simulink model "ModeShape_IEEE14_case1"  (R2022b)
settings: Solver=FixedStepAuto  StartTime=0.0  StopTime=15  FixedStep=Ts  RelTol=1e-3
InitFcn:
  | load('data_idq_all');
  | load('data_vdq_all');
  | ModeSel = 151; % case1
  | run Mode_Right_Eig.m;
StartFcn:
  | load('data_idq_all');
  | load('data_vdq_all');
  | ModeSel = 151; % case1
  | run Mode_Right_Eig.m;
values from neighbouring files (symbols this model uses):
  freq_sel = imag(Mode_Hz)    [Mode_Right_Eig.m]
  Mode_Rad = D(ModeSel, ModeSel)    [Mode_Right_Eig.m]
  Phi_vec_trim = Phi_vec_trim.'    [Mode_Right_Eig.m]
  Psi_vec_trim = Psi_vec_trim.'    [Mode_Right_Eig.m]
undefined symbols (not defined in the file or in its folder): Ts
libraries: eeGeneralControl x4, spsPLLLib x1
settings Model: Creator=y_zhu  LastModifiedBy=yz34218

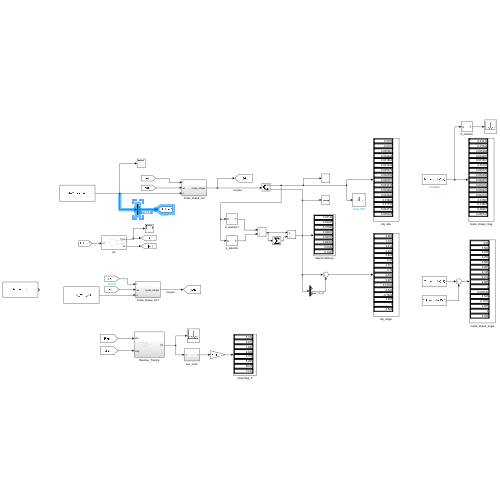
[thumbnail: Simulink's stored preview of the top-level diagram]
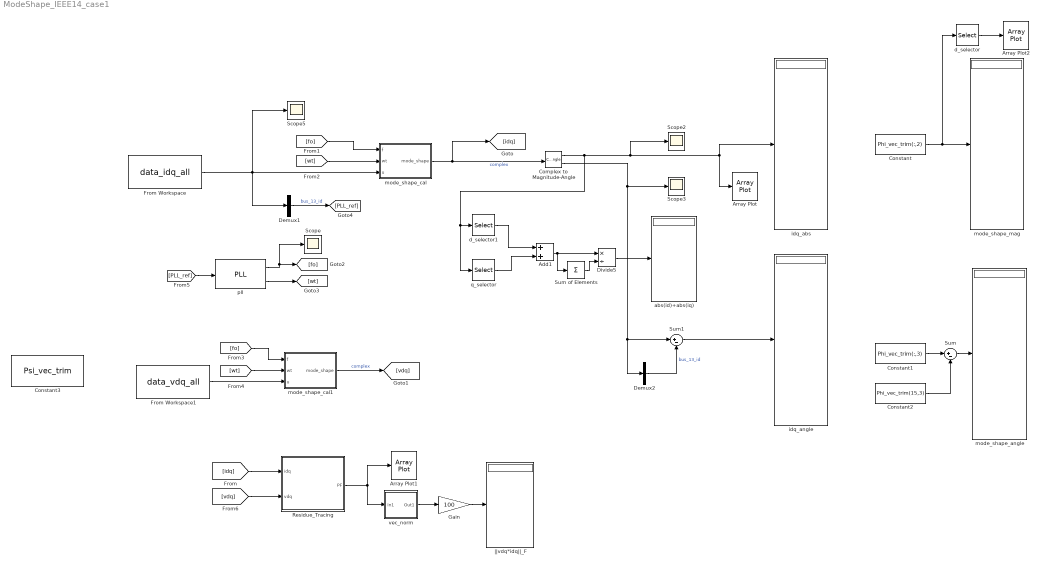
== system ModeShape_IEEE14_case1 ==
  Add1 : Sum
  Array Plot : ArrayPlot  WindowPosition=[-4.000000,155.000000,800.000000,500.000000,]  ScopeFrameLocation=window  YLimits=[-0.001,0.0195]
  Array Plot1 : ArrayPlot  WindowPosition=[913.000000,343.000000,800.000000,500.000000,]  ScopeFrameLocation=window  YLimits=[-0.0628,0.6743]
  Array Plot2 : ArrayPlot  WindowPosition=[402.000000,155.000000,800.000000,621.000000,]  ScopeFrameLocation=window  YLimits=[-0.0001,0.018]
  Complex to Magnitude-Angle : ComplexToMagnitudeAngle
  Constant : Constant  Value=Phi_vec_trim(:,2)
  Constant1 : Constant  Value=Phi_vec_trim(:,3)
  Constant2 : Constant  Value=Phi_vec_trim(15,3)
  Constant3 : Constant  Value=Psi_vec_trim
  Demux1 : Demux  Outputs=[14,1,1]
  Demux2 : Demux  Outputs=[14,1,1]
  Divide5 : Product  Inputs=*/
  From Workspace : FromWorkspace  VariableName=data_idq_all
  From Workspace1 : FromWorkspace  VariableName=data_vdq_all
  Gain : Gain  Gain=100
  Residue_Tracing : Subsystem
  Scope{,2..3,5} (4 alike) : Scope
  Sum : Sum  Inputs=|+-
  Sum of Elements : Sum  Inputs=+
  Sum1 : Sum  Inputs=|+-
  abs(id)+abs(iq) : Display
  d_selector : Selector  InputPortWidth=length(Phi_vec_trim)  IndexOptions=Index vector (dialog)  Indices=[1:2:length(Phi_vec_trim)]  OutputSizes=1
  d_selector1 : Selector  InputPortWidth=length(Phi_vec_trim)  IndexOptions=Index vector (dialog)  Indices=[1:2:length(Phi_vec_trim)]  OutputSizes=1
  idq_abs : Display
  idq_angle : Display
  mode_shape_angle : Display
  mode_shape_cal : Subsystem
  mode_shape_cal1 : Subsystem
  mode_shape_mag : Display
  pll : spsPLLLib/PLL  Fmin=freq_sel/2  Par_Init=[0, freq_sel]  ParK=[50, 200, 1]  TcD=Ts*10  MaxRateChangeFreq=1  FilterCutOffFreq=4  Ts=Ts*10  AGC=on
      settings: LibrarySourceBlock=sps_lib/Control/PLL
  q_selector : Selector  InputPortWidth=length(Phi_vec_trim)  IndexOptions=Index vector (dialog)  Indices=[2:2:length(Phi_vec_trim)]  OutputSizes=1
  vec_norm : Subsystem
  ||vdq*idq||_F : Display
  wires:
  From Workspace/1 -> Demux1/1, Scope5/1, mode_shape_cal/3(u)
  pll/1 -> [fo], Scope/1
  pll/2 -> [wt]
  Constant/1 -> mode_shape_mag/1, d_selector/1
  Constant1/1 -> Sum/1
  Constant2/1 -> Sum/2
  [fo] -> mode_shape_cal/1(f)
  [wt] -> mode_shape_cal/2(wt)
  mode_shape_cal/1(mode_shape) -> Complex to Magnitude-Angle/1, [idq]  "complex"
  Demux1/2 -> [PLL_ref]  "bus_13_id"
  Complex to Magnitude-Angle/2 -> Scope3/1, Demux2/1, Sum1/1
  Demux2/2 -> Sum1/2  "bus_13_id"
  [wt] -> mode_shape_cal1/2(wt)
  [fo] -> mode_shape_cal1/1(f)
  From Workspace1/1 -> mode_shape_cal1/3(u)
  Complex to Magnitude-Angle/1 -> q_selector/1, d_selector1/1, Array Plot/1, idq_abs/1, Scope2/1
  d_selector1/1 -> Add1/1
  mode_shape_cal1/1(mode_shape) -> [vdq]  "complex"
  Sum/1 -> mode_shape_angle/1
  Sum1/1 -> idq_angle/1
  Add1/1 -> Divide5/1, Sum of Elements/1
  Sum of Elements/1 -> Divide5/2
  Divide5/1 -> abs(id)+abs(iq)/1
  q_selector/1 -> Add1/2
  [idq] -> Residue_Tracing/1(idq)
  [vdq] -> Residue_Tracing/2(vdq)
  Residue_Tracing/1(PF) -> Array Plot1/1, vec_norm/1(In1)
  d_selector/1 -> Array Plot2/1
  Gain/1 -> ||vdq*idq||_F/1
  vec_norm/1(Out1) -> Gain/1
  [PLL_ref] -> pll/1

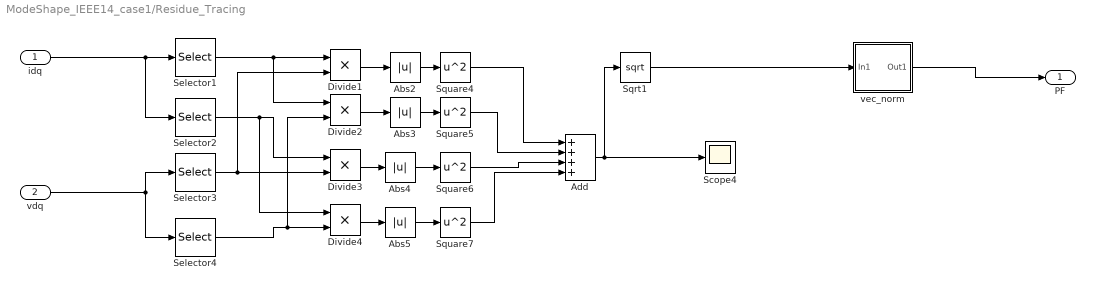
== system ModeShape_IEEE14_case1/Residue_Tracing ==
  idq : Inport
  vdq : Inport  Port=2
  Abs{2..5} (4 alike) : Abs  SaturateOnIntegerOverflow=off
  Add : Sum  Inputs=++++
  Divide{1..4} (4 alike) : Product  Inputs=**
  Scope4 : Scope
  Selector1 : Selector  InputPortWidth=16  IndexOptions=Index vector (dialog)  Indices=[1:2:15]  OutputSizes=1
  Selector2 : Selector  InputPortWidth=16  IndexOptions=Index vector (dialog)  Indices=[2:2:16]  OutputSizes=1
  Selector3 : Selector  InputPortWidth=16  IndexOptions=Index vector (dialog)  Indices=[1:2:15]  OutputSizes=1
  Selector4 : Selector  InputPortWidth=16  IndexOptions=Index vector (dialog)  Indices=[2:2:16]  OutputSizes=1
  Sqrt1 : Sqrt
  Square{4..7} (4 alike) : Math  Operator=square
  vec_norm : Subsystem
  PF : Outport
  wires:
  Selector2/1 -> Divide4/1, Divide3/1
  Square6/1 -> Add/3
  Selector4/1 -> Divide2/2, Divide4/2
  Divide1/1 -> Abs2/1
  vdq/1 -> Selector4/1, Selector3/1
  idq/1 -> Selector2/1, Selector1/1
  Selector1/1 -> Divide2/1, Divide1/1
  Abs5/1 -> Square7/1
  Divide2/1 -> Abs3/1
  Selector3/1 -> Divide3/2, Divide1/2
  Divide4/1 -> Abs5/1
  Divide3/1 -> Abs4/1
  Abs2/1 -> Square4/1
  Add/1 -> Scope4/1, Sqrt1/1
  Abs4/1 -> Square6/1
  Abs3/1 -> Square5/1
  Square4/1 -> Add/1
  Square5/1 -> Add/2
  Square7/1 -> Add/4
  Sqrt1/1 -> vec_norm/1(In1)
  vec_norm/1(Out1) -> PF/1

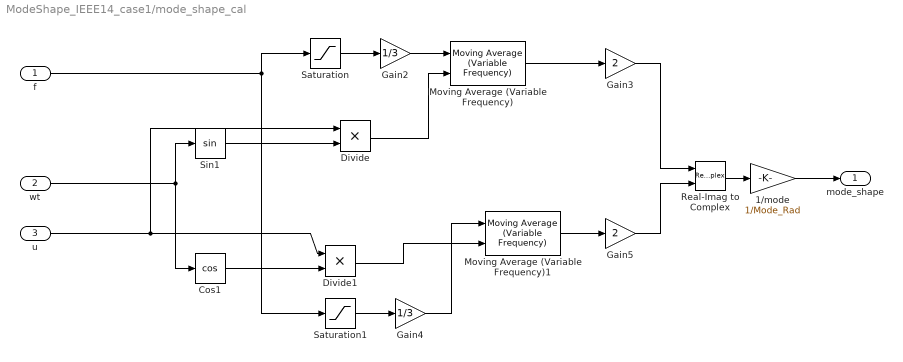
== system ModeShape_IEEE14_case1/mode_shape_cal ==
  f : Inport
  wt : Inport  Port=2
  u : Inport  Port=3
  1/mode : Gain  Gain=1/Mode_Rad
  Cos1 : Trigonometry  Operator=cos
  Divide : Product  Inputs=**
  Divide1 : Product  Inputs=**
  Gain2 : Gain  Gain=1/3
  Gain3 : Gain  Gain=2
  Gain4 : Gain  Gain=1/3
  Gain5 : Gain  Gain=2
  Moving Average (Variable Frequency) : eeGeneralControl/Moving Average (Variable Frequency)  VariantControl=Variant1  LabelModeActiveChoice=Discrete  f0=2  fmin=0.1  x0=0  BufferSize=8192  Ts=Ts*100
      settings: LibrarySourceBlock=|
      | ee_sl_lib/General Control/Moving Average
      | (Variable Frequency)
  Moving Average (Variable Frequency)1 : eeGeneralControl/Moving Average (Variable Frequency)  VariantControl=Variant1  LabelModeActiveChoice=Discrete  f0=2  fmin=0.1  x0=0  BufferSize=8192  Ts=Ts*100
      settings: LibrarySourceBlock=|
      | ee_sl_lib/General Control/Moving Average
      | (Variable Frequency)
  Real-Imag to Complex : RealImagToComplex
  Saturation : Saturate  UpperLimit=9  LowerLimit=8.5
  Saturation1 : Saturate  UpperLimit=9  LowerLimit=8.5
  Sin1 : Trigonometry
  mode_shape : Outport
  wires:
  wt/1 -> Cos1/1, Sin1/1
  Divide1/1 -> Moving Average (Variable Frequency)1/2
  Cos1/1 -> Divide1/2
  Saturation1/1 -> Gain4/1
  Moving Average (Variable Frequency)1/1 -> Gain5/1
  Saturation/1 -> Gain2/1
  Gain2/1 -> Moving Average (Variable Frequency)/1
  f/1 -> Saturation/1, Saturation1/1
  Gain4/1 -> Moving Average (Variable Frequency)1/1
  Divide/1 -> Moving Average (Variable Frequency)/2
  Real-Imag to Complex/1 -> 1/mode/1
  Gain3/1 -> Real-Imag to Complex/1
  Gain5/1 -> Real-Imag to Complex/2
  u/1 -> Divide1/1, Divide/1
  Moving Average (Variable Frequency)/1 -> Gain3/1
  Sin1/1 -> Divide/2
  1/mode/1 -> mode_shape/1

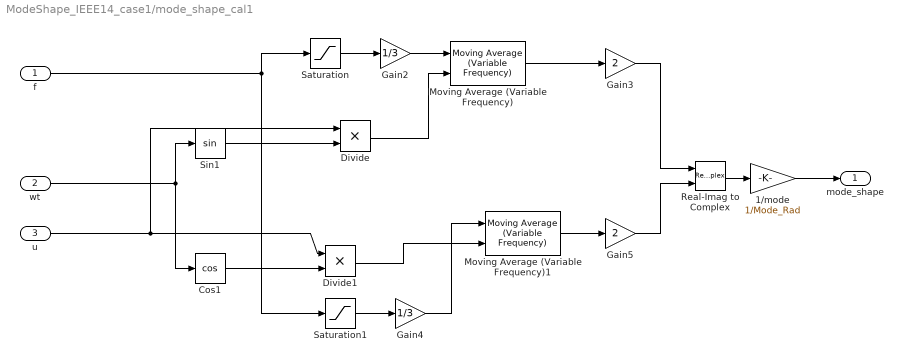
== system ModeShape_IEEE14_case1/mode_shape_cal1 ==
  f : Inport
  wt : Inport  Port=2
  u : Inport  Port=3
  1/mode : Gain  Gain=1/Mode_Rad
  Cos1 : Trigonometry  Operator=cos
  Divide : Product  Inputs=**
  Divide1 : Product  Inputs=**
  Gain2 : Gain  Gain=1/3
  Gain3 : Gain  Gain=2
  Gain4 : Gain  Gain=1/3
  Gain5 : Gain  Gain=2
  Moving Average (Variable Frequency) : eeGeneralControl/Moving Average (Variable Frequency)  VariantControl=Variant1  LabelModeActiveChoice=Discrete  f0=2  fmin=0.1  x0=0  BufferSize=8192  Ts=Ts*100
      settings: LibrarySourceBlock=|
      | ee_sl_lib/General Control/Moving Average
      | (Variable Frequency)
  Moving Average (Variable Frequency)1 : eeGeneralControl/Moving Average (Variable Frequency)  VariantControl=Variant1  LabelModeActiveChoice=Discrete  f0=2  fmin=0.1  x0=0  BufferSize=8192  Ts=Ts*100
      settings: LibrarySourceBlock=|
      | ee_sl_lib/General Control/Moving Average
      | (Variable Frequency)
  Real-Imag to Complex : RealImagToComplex
  Saturation : Saturate  UpperLimit=9  LowerLimit=8.5
  Saturation1 : Saturate  UpperLimit=9  LowerLimit=8.5
  Sin1 : Trigonometry
  mode_shape : Outport
  wires:
  wt/1 -> Cos1/1, Sin1/1
  Divide1/1 -> Moving Average (Variable Frequency)1/2
  Cos1/1 -> Divide1/2
  Saturation1/1 -> Gain4/1
  Moving Average (Variable Frequency)1/1 -> Gain5/1
  Saturation/1 -> Gain2/1
  Gain2/1 -> Moving Average (Variable Frequency)/1
  f/1 -> Saturation/1, Saturation1/1
  Gain4/1 -> Moving Average (Variable Frequency)1/1
  Divide/1 -> Moving Average (Variable Frequency)/2
  Real-Imag to Complex/1 -> 1/mode/1
  Gain3/1 -> Real-Imag to Complex/1
  Gain5/1 -> Real-Imag to Complex/2
  u/1 -> Divide1/1, Divide/1
  Moving Average (Variable Frequency)/1 -> Gain3/1
  Sin1/1 -> Divide/2
  1/mode/1 -> mode_shape/1

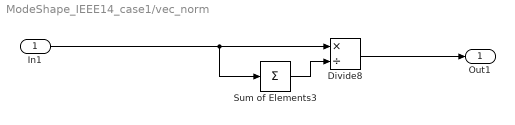
== system ModeShape_IEEE14_case1/vec_norm ==
  In1 : Inport
  Divide8 : Product  Inputs=*/
  Sum of Elements3 : Sum  Inputs=+
  Out1 : Outport
  wires:
  Sum of Elements3/1 -> Divide8/2
  In1/1 -> Sum of Elements3/1, Divide8/1
  Divide8/1 -> Out1/1

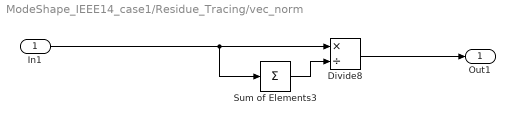
== system ModeShape_IEEE14_case1/Residue_Tracing/vec_norm ==
  In1 : Inport
  Divide8 : Product  Inputs=*/
  Sum of Elements3 : Sum  Inputs=+
  Out1 : Outport
  wires:
  Sum of Elements3/1 -> Divide8/2
  In1/1 -> Sum of Elements3/1, Divide8/1
  Divide8/1 -> Out1/1
